simulink model "Control_test"  (R2014b)
settings: Solver=FixedStepDiscrete  StartTime=0.0  StopTime=Inf  FixedStep=0.001  RelTol=1e-3
PostLoadFcn:
  | , if any(exist('dsrtsu_mdlpostloadfcn', 'file') == [2, 3, 6]), try dsrtsu_mdlpostloadfcn('Execute', bdroot); catch fprintf('Error in PostLoadFcn (dsrtsu_mdlpostloadfcn) for model "%s":\n %s\n', bdroot, lasterr); end, end,
undefined symbols (not defined in the file or in its folder): dtLocal, slcm
libraries: rtican x163, simulink x14
(part 30 of 34)

== system Control_test/InputProcessing/RadarCanProcessing/Track64 ==
  Bus Creator : BusCreator  Inputs=12
  ESR_Track64 : rtican/RTICAN Receive (RX)   Reserved1=[]  Reserved2=[]  Reserved3=[]  Reserved4=[]  SfcnMessage=[]  Msg_Struct=[]  BoardTypeNo=[]  BoardNo=[]  ChannelNo=[]  Parameters=[]  DialogFcn=[]  UnitName=[]  Revision=[]  UnitValues=[]  DSProperties=struct('RTI',struct('Version',uint32(5),'BlockType',struct('isSLSource',uint8(1),'isSLSink',uint8(1),'isHWSource',uint8(0),'isHWSink',uint8(0),'isSetup',uint8(0),'isInline',uint8(1),'isNonInline',uint8(0),'isInterrupt',uint8(0),'isChannelwise',uint8(0)),'IOBoardType','RTICAN','UnitType','MESSAGE','Identifier','RX','DialogType','MSVC','BlockSet','RTICAN','SlaveProcessor','CAN'))  RTIBlockInterface=struct('OutputPortsWidth',int32([1 1 1 1 1 1 1 1 1 1 1 1]),'OutputPortsActive',[1 1 1 1 1 1 1 1 1 1 1 1],'OutputPortsName',{{'CAN_TX_TRACK_RANGE_RATE_64','CAN_TX_TRACK_MED_RANGE_MODE_64','CAN_TX_TRACK_RANGE_ACCEL_64','CAN_TX_TRACK_WIDTH_64','CAN_TX_TRACK_ROLLING_COUNT_64','CAN_TX_TRACK_BRIDGE_OBJECT_64','CAN_TX_TRACK_RANGE_64','CAN_TX_TRACK_ANGLE_64','CAN_TX_TRACK_STATUS_64','CAN_TX_TRACK_ONCOMING_64','CAN_TX_TRACK_GROUPING_CHANGED_64','CAN_TX_TRACK_LAT_RATE_64'}},'OutputPortsDataType',{{'SS_DOUBLE','SS_DOUBLE','SS_DOUBLE','SS_DOUBLE','SS_DOUBLE','SS_DOUBLE','SS_DOUBLE','SS_DOUBLE','SS_DOUBLE','SS_DOUBLE','SS_DOUBLE','SS_DOUBLE'}},'OutputPortsLabel',{{'CAN_TX_TRACK_RANGE_RATE_64','CAN_TX_TRACK_MED_RANGE_MODE_64','CAN_TX_TRACK_RANGE_ACCEL_64','CAN_TX_TRACK_WIDTH_64','CAN_TX_TRACK_ROLLING_COUNT_64','CAN_TX_TRACK_BRIDGE_OBJECT_64','CAN_TX_TRACK_RANGE_64','CAN_TX_TRACK_ANGLE_64','CAN_TX_TRACK_STATUS_64','CAN_TX_TRACK_ONCOMING_64','CAN_TX_TRACK_GROUPING_CHANGED_64','CAN_TX_TRACK_LAT_RATE_64'}},'OutputPortsLabelMode','ON','InputPortsWidth',int32(0),'InputPortsActive',0,'DialogFcn','rtican_message_interface_gui','BlockDisplay',{{'','center'}},'IconTransparency','on','ParameterTunableNames',{{}},'InitLevel',3,'BlockName',struct('Token',{{'ESR_Track64'}}),'SampleTime',{{0.01}},'TriggerPort',{{'none'}},'EnablePort',{{'none'}})  RTIBlockParameters=struct('BoardTypeNo',{{1,'OFF',[]}},'BoardNo',{{2,'ON',[1 16]}},'ChannelNo',{{2,'ON',[1 2]}},'Parameters',{{struct('DataFileSupport',struct('DataFileSelectedMaster',1,'DataFileSelectedLocal',0,'DataFileName','c:\users\mpc_car\documents\github\mpc-car\controller\dbcfiles\esr_dv3_64tgt.dbc|','DataFileDate',{{{['02-Nov-2012 20:32:52']},{['21-Mar-2013 13:39:53']},{['28-Sep-2011 17:08:52']}}},'SelectedFile',['<no file selected>'],'InterfaceFcn','rtican_dbc_file_parser'),'Options',struct('StatusSelected',0,'TimeSelected',0,'DeltaTimeSelected',0,'BytePortSelected',0,'MessageLengthSelected',0,'TriggerPort',struct('Selected',0,'TriggerType',0),'UserCoding',struct('Selected',0,'InterfaceFile','UserDecodingFile','FcnName','UserDecodeFcn','InportSelected',0,'InportWidth',1,'OutportSelected',0,'OutportWidth',1),'EnablePortSelected',0,'SignalOnPortnameSelected',1,'UseRXService',0),'Message',struct('MsgOnBlocknameSelected',1,'MsgName','ESR_Track64','MsgIdFormat',0,'MsgId',1343,'MsgLength',8,'NumSignals',12,'SampleTime',0.01,'Signal',struct('SgnName',{'CAN_TX_TRACK_RANGE_RATE_64','CAN_TX_TRACK_MED_RANGE_MODE_64','CAN_TX_TRACK_RANGE_ACCEL_64','CAN_TX_TRACK_WIDTH_64','CAN_TX_TRACK_ROLLING_COUNT_64','CAN_TX_TRACK_BRIDGE_OBJECT_64','CAN_TX_TRACK_RANGE_64','CAN_TX_TRACK_ANGLE_64','CAN_TX_TRACK_STATUS_64','CAN_TX_TRACK_ONCOMING_64','CAN_TX_TRACK_GROUPING_CHANGED_64','CAN_TX_TRACK_LAT_RATE_64'},'SgnStartBit',{0,14,16,26,30,31,32,43,53,56,57,58},'SgnLength',{14,2,10,4,1,1,11,10,3,1,1,6},'SgnType',{0,0,0,0,0,0,0,0,0,0,0,0},'ModeValue',{-1,-1,-1,-1,-1,-1,-1,-1,-1,-1,-1,-1},'DataType',{1,0,1,0,0,0,0,1,0,0,0,1},'ByteLayout',{2,2,2,2,2,2,2,2,2,2,2,2},'Factor',{0.01,1,0.05,0.5,1,1,0.1,0.1,1,1,1,0.25},'Offset',{0,0,0,0,0,0,0,0,0,0,0,0},'SgnComment',{{''},{''},{''},{''},{''},{''},{''},{''},{''},{''},{''},{''}},'SgnUnit',{'m/s','','m/s/s','m','','','m','deg','','','',''},'Min',{-81.92,0,-25.6,0,0,0,0,-51.2,0,0,0,-8},'Max',{81.91,3,25.55,7.5,1,0,204.7,51.1,7,0,0,7.75},'SLDataType',{'SS_DOUBLE','SS_DOUBLE','SS_DOUBLE','SS_DOUBLE','SS_DOUBLE','SS_DOUBLE','SS_DOUBLE','SS_DOUBLE','SS_DOUBLE','SS_DOUBLE','SS_DOUBLE','SS_DOUBLE'}),'MsgIdNumFormat',0,'MsgComment',{{''}}),'Version',1.2,'general',struct('isFromLib',0)),'OFF',[]}},'GroupId',{{struct('Group',{{'RTICAN'}},'No',4,'Behavior',{{'NAMECHANGE'}},'BlockType',{{'SINK'}},'NameChangeFlag',0),'OFF',[]}},'SFcnRTICANMessage',{{struct('MsgType','RX','SFcnPortType','Scalar','MsgName','ESR_Track64','MsgIdFormat','STD','MsgId',1343,'MsgLength',8,'NumSignals',12,'SampleTime',0.01,'Signal',struct('SgnName',{'CAN_TX_TRACK_RANGE_RATE_64','CAN_TX_TRACK_MED_RANGE_MODE_64','CAN_TX_TRACK_RANGE_ACCEL_64','CAN_TX_TRACK_WIDTH_64','CAN_TX_TRACK_ROLLING_COUNT_64','CAN_TX_TRACK_BRIDGE_OBJECT_64','CAN_TX_TRACK_RANGE_64','CAN_TX_TRACK_ANGLE_64','CAN_TX_TRACK_STATUS_64','CAN_TX_TRACK_ONCOMING_64','CAN_TX_TRACK_GROUPING_CHANGED_64','CAN_TX_TRACK_LAT_RATE_64'},'SgnStartBit',{0,14,16,26,30,31,32,43,53,56,57,58},'SgnLength',{14,2,10,4,1,1,11,10,3,1,1,6},'SgnType',{'standard','standard','standard','standard','standard','standard','standard','standard','standard','standard','standard','standard'},'ModeValue',{-1,-1,-1,-1,-1,-1,-1,-1,-1,-1,-1,-1},'DataType',{['signed int'],['unsigned int'],['signed int'],['unsigned int'],['unsigned int'],['unsigned int'],['unsigned int'],['signed int'],['unsigned int'],['unsigned int'],['unsigned int'],['signed int']},'ByteLayout',{['motorola back.'],['motorola back.'],['motorola back.'],['motorola back.'],['motorola back.'],['motorola back.'],['motorola back.'],['motorola back.'],['motorola back.'],['motorola back.'],['motorola back.'],['motorola back.']},'Factor',{0.01,1,0.05,0.5,1,1,0.1,0.1,1,1,1,0.25},'Offset',{0,0,0,0,0,0,0,0,0,0,0,0},'SLDataType',{'SS_DOUBLE','SS_DOUBLE','SS_DOUBLE','SS_DOUBLE','SS_DOUBLE','SS_DOUBLE','SS_DOUBLE','SS_DOUBLE','SS_DOUBLE','SS_DOUBLE','SS_DOUBLE','SS_DOUBLE'}),'StatusSelected','no','TimeSelected','no','DeltaTimeSelected','no','BytePortSelected','no','MessageLengthSelected','no','TriggerPort',struct('Selected','no','TriggerType',0),'UserCoding',struct('Selected','no','InterfaceFile','UserDecodingFile','FcnName','UserDecodeFcn','InportSelected','no','InportWidth',1,'OutportSelected','no','OutportWidth',1),'EnablePortSelected','no','UseRXService','no','BoardType','DS1','BoardNo',2,'ControllerNo',2),'OFF',[]}},'TLCFileName',{{'rtican_rx_message','OFF',[]}})  RTISFcnParameters=struct('SFcnRTICANMessage','struct','TLCFileName','char')  RTIBlockParaDefault=struct('BoardTypeNo',4302,'BoardNo',1,'ChannelNo',1,'Parameters',struct('DataFileSupport',struct('DataFileSelectedMaster',0,'DataFileSelectedLocal',0,'DataFileName','','DataFileDate','','SelectedFile',['<no file selected>']),'Options',struct('StatusSelected',1,'TimeSelected',1,'DeltaTimeSelected',1,'BytePortSelected',0,'MessageLengthSelected',0,'TriggerPort',struct('Selected',0,'TriggerType','rising'),'UserCoding',struct('Selected',0,'InterfaceFile','UserDecodingFile','FcnName','UserDecodeFcn','InportSelected',0,'InportWidth',1,'OutportSelected',0,'OutportWidth',1),'EnablePortSelected',0,'SignalOnPortnameSelected',1,'UseRXService',0),'Message',struct('MsgOnBlocknameSelected',0,'MsgName',['RX Message'],'MsgIdFormat',0,'MsgId',100,'MsgLength',8,'NumSignals',1,'SampleTime',-1,'Signal',struct('SgnName',['RX signal'],'SgnStartBit',0,'SgnLength',8,'SgnType',0,'ModeValue',-1,'DataType',0,'SLDataType','SS_DOUBLE','ByteLayout',0,'Factor',1,'Offset',0,'Min',0,'Max',255,'SgnComment',{{}},'SgnUnit',''),'MsgIdNumFormat',0,'MsgComment',{{''}}),'Version',1.2,'general',struct('isFromLib',1)),'GroupId',struct('Group',{{'RTICAN'}},'No',1,'Behavior',{{'NAMECHANGE'}},'BlockType',{{'SINK'}},'NameChangeFlag',0),'SFcnRTICANMessage',struct('MsgType','RX','MsgName',['RX Message'],'MsgIdFormat','STD','MsgId',100,'MsgLength',8,'NumSignals',1,'SampleTime',-1,'Signal',struct('SgnName',['RX signal'],'SgnStartBit',0,'SgnLength',8,'SgnType','standard','ModeValue',-1,'DataType',['unsigned int'],'ByteLayout',['little endian'],'SLDataType','SS_DOUBLE','Factor',1,'Offset',0),'StatusSelected','yes','TimeSelected','yes','DeltaTimeSelected','yes','BytePortSelected','no','MessageLengthSelected','no','EnablePortSelected','no','UserCoding',struct('Selected','no','InterfaceFile','UserDecodingFile','FcnName','UserDecodeFcn','InportSelected','no','InportWidth',1,'OutportSelected','no','OutportWidth',1),'TriggerPort',struct('Selected','no','TriggerType','rising'),'UseRXService','no','BoardType','DS4302','BoardNo',1,'ControllerNo',1,'SFcnPortType','Scalar'),'TLCFileName','rtican_rx_message')
      settings: AttributesFormatString=Group Id: RTICAN4\n
  Out1 : Outport
  wires:
  Bus Creator/1 -> Out1/1  "Track64"
  ESR_Track64/1 -> Bus Creator/1  "CAN_TX_TRACK_RANGE_RATE_64"
  ESR_Track64/2 -> Bus Creator/2  "CAN_TX_TRACK_MED_RANGE_MODE_64"
  ESR_Track64/3 -> Bus Creator/3  "CAN_TX_TRACK_RANGE_ACCEL_64"
  ESR_Track64/4 -> Bus Creator/4  "CAN_TX_TRACK_WIDTH_64"
  ESR_Track64/5 -> Bus Creator/5  "CAN_TX_TRACK_ROLLING_COUNT_64"
  ESR_Track64/6 -> Bus Creator/6  "CAN_TX_TRACK_BRIDGE_OBJECT_64"
  ESR_Track64/7 -> Bus Creator/7  "CAN_TX_TRACK_RANGE_64"
  ESR_Track64/8 -> Bus Creator/8  "CAN_TX_TRACK_ANGLE_64"
  ESR_Track64/9 -> Bus Creator/9  "CAN_TX_TRACK_STATUS_64"
  ESR_Track64/10 -> Bus Creator/10  "CAN_TX_TRACK_ONCOMING_64"
  ESR_Track64/11 -> Bus Creator/11  "CAN_TX_TRACK_GROUPING_CHANGED_64"
  ESR_Track64/12 -> Bus Creator/12  "CAN_TX_TRACK_LAT_RATE_64"

== system Control_test/InputProcessing/VehicleCanProcessing/CLU1 ==
  Bus Creator : BusCreator  Inputs=15
  L_CLU1 : rtican/RTICAN Receive (RX)   Reserved1=[]  Reserved2=[]  Reserved3=[]  Reserved4=[]  SfcnMessage=[]  Msg_Struct=[]  BoardTypeNo=[]  BoardNo=[]  ChannelNo=[]  Parameters=[]  DialogFcn=[]  UnitName=[]  Revision=[]  UnitValues=[]  DSProperties=struct('RTI',struct('Version',uint32(5),'BlockType',struct('isSLSource',uint8(1),'isSLSink',uint8(1),'isHWSource',uint8(0),'isHWSink',uint8(0),'isSetup',uint8(0),'isInline',uint8(1),'isNonInline',uint8(0),'isInterrupt',uint8(0),'isChannelwise',uint8(0)),'IOBoardType','RTICAN','UnitType','MESSAGE','Identifier','RX','DialogType','MSVC','BlockSet','RTICAN','SlaveProcessor','CAN'))  RTIBlockInterface=struct('OutputPortsWidth',int32([1 1 1 1 1 1 1 1 1 1 1 1 1 1 1]),'OutputPortsActive',[1 1 1 1 1 1 1 1 1 1 1 1 1 1 1],'OutputPortsName',{{'CruiseSWStatus','CF_Blr_MaxStat','CF_Clu_SldMainSW','SPEED_UNIT','P_Brake_ACT','Vanz','AliveCounter','CruiseSW_Main','DashACCFail','DISFail','VEHICLE_INFO','CF_StrRly_Stat','CF_ButSys_VarInd','R_TqAcnOutC','Odometer'}},'OutputPortsDataType',{{'SS_DOUBLE','SS_DOUBLE','SS_DOUBLE','SS_DOUBLE','SS_DOUBLE','SS_DOUBLE','SS_DOUBLE','SS_DOUBLE','SS_DOUBLE','SS_DOUBLE','SS_DOUBLE','SS_DOUBLE','SS_DOUBLE','SS_DOUBLE','SS_DOUBLE'}},'OutputPortsLabel',{{'CruiseSWStatus','CF_Blr_MaxStat','CF_Clu_SldMainSW','SPEED_UNIT','P_Brake_ACT','Vanz','AliveCounter','CruiseSW_Main','DashACCFail','DISFail','VEHICLE_INFO','CF_StrRly_Stat','CF_ButSys_VarInd','R_TqAcnOutC','Odometer'}},'OutputPortsLabelMode','ON','InputPortsWidth',int32(0),'InputPortsActive',0,'DialogFcn','rtican_message_interface_gui','BlockDisplay',{{'','center'}},'IconTransparency','on','ParameterTunableNames',{{}},'InitLevel',3,'BlockName',struct('Token',{{'L_CLU1'}}),'SampleTime',{{-1}},'TriggerPort',{{'none'}},'EnablePort',{{'none'}})  RTIBlockParameters=struct('BoardTypeNo',{{1,'OFF',[]}},'BoardNo',{{1,'ON',[1 16]}},'ChannelNo',{{1,'ON',[1 2]}},'Parameters',{{struct('DataFileSupport',struct('DataFileSelectedMaster',1,'DataFileSelectedLocal',1,'DataFileName','c:\users\mpc_car\documents\github\mpc-car\controller\dbcfiles\hmc_can_for_ucb_v2.dbc|','DataFileDate',{{{['21-Nov-2014 13:30:51']}}},'SelectedFile','c:\users\mpc_car\documents\github\mpc-car\dbcfiles\hmc_can_for_ucb_v2.dbc','InterfaceFcn','rtican_dbc_file_parser'),'Options',struct('StatusSelected',0,'TimeSelected',0,'DeltaTimeSelected',0,'BytePortSelected',0,'MessageLengthSelected',0,'TriggerPort',struct('Selected',0,'TriggerType',0),'UserCoding',struct('Selected',0,'InterfaceFile','UserDecodingFile','FcnName','UserDecodeFcn','InportSelected',0,'InportWidth',1,'OutportSelected',0,'OutportWidth',1),'EnablePortSelected',0,'SignalOnPortnameSelected',1,'UseRXService',0),'Message',struct('MsgOnBlocknameSelected',1,'MsgName','L_CLU1','MsgIdFormat',0,'MsgId',1264,'MsgLength',8,'NumSignals',15,'SampleTime',-1,'Signal',struct('SgnName',{'CruiseSWStatus','CF_Blr_MaxStat','CF_Clu_SldMainSW','SPEED_UNIT','P_Brake_ACT','Vanz','AliveCounter','CruiseSW_Main','DashACCFail','DISFail','VEHICLE_INFO','CF_StrRly_Stat','CF_ButSys_VarInd','R_TqAcnOutC','Odometer'},'SgnStartBit',{0,3,4,6,7,8,17,24,25,26,27,30,31,32,40},'SgnLength',{3,1,1,1,1,9,7,1,1,1,3,1,1,8,24},'SgnType',{0,0,0,0,0,0,0,0,0,0,0,0,0,0,0},'ModeValue',{-1,-1,-1,-1,-1,-1,-1,-1,-1,-1,-1,-1,-1,-1,-1},'DataType',{0,0,0,0,0,0,0,0,0,0,0,0,0,0,0},'ByteLayout',{0,0,0,0,0,0,0,0,0,0,0,0,0,0,0},'Factor',{1,1,1,1,1,1,1,1,1,1,1,1,1,1,1},'Offset',{0,0,0,0,0,0,0,0,0,0,0,0,0,0,0},'SgnComment',{{''},{''},{''},{''},{''},{''},{''},{''},{''},{''},{''},{''},{''},{''},{''}},'SgnUnit',{'','','','','',['km/h or MPH'],'','','','','','','','Nm','km'},'Min',{0,0,0,0,0,0,0,0,0,0,0,0,0,0,0},'Max',{7,1,1,1,1,255.5,127,1,1,1,7,1,1,255,1677721.5},'SLDataType',{'SS_DOUBLE','SS_DOUBLE','SS_DOUBLE','SS_DOUBLE','SS_DOUBLE','SS_DOUBLE','SS_DOUBLE','SS_DOUBLE','SS_DOUBLE','SS_DOUBLE','SS_DOUBLE','SS_DOUBLE','SS_DOUBLE','SS_DOUBLE','SS_DOUBLE'}),'MsgIdNumFormat',0,'MsgComment',{{''}}),'Version',1.2,'general',struct('isFromLib',0)),'OFF',[]}},'GroupId',{{struct('Group',{{'RTICAN'}},'No',1,'Behavior',{{'NAMECHANGE'}},'BlockType',{{'SINK'}},'NameChangeFlag',0),'OFF',[]}},'SFcnRTICANMessage',{{struct('MsgType','RX','SFcnPortType','Scalar','MsgName','L_CLU1','MsgIdFormat','STD','MsgId',1264,'MsgLength',8,'NumSignals',15,'SampleTime',-1,'Signal',struct('SgnName',{'CruiseSWStatus','CF_Blr_MaxStat','CF_Clu_SldMainSW','SPEED_UNIT','P_Brake_ACT','Vanz','AliveCounter','CruiseSW_Main','DashACCFail','DISFail','VEHICLE_INFO','CF_StrRly_Stat','CF_ButSys_VarInd','R_TqAcnOutC','Odometer'},'SgnStartBit',{0,3,4,6,7,8,17,24,25,26,27,30,31,32,40},'SgnLength',{3,1,1,1,1,9,7,1,1,1,3,1,1,8,24},'SgnType',{'standard','standard','standard','standard','standard','standard','standard','standard','standard','standard','standard','standard','standard','standard','standard'},'ModeValue',{-1,-1,-1,-1,-1,-1,-1,-1,-1,-1,-1,-1,-1,-1,-1},'DataType',{['unsigned int'],['unsigned int'],['unsigned int'],['unsigned int'],['unsigned int'],['unsigned int'],['unsigned int'],['unsigned int'],['unsigned int'],['unsigned int'],['unsigned int'],['unsigned int'],['unsigned int'],['unsigned int'],['unsigned int']},'ByteLayout',{['little endian'],['little endian'],['little endian'],['little endian'],['little endian'],['little endian'],['little endian'],['little endian'],['little endian'],['little endian'],['little endian'],['little endian'],['little endian'],['little endian'],['little endian']},'Factor',{1,1,1,1,1,1,1,1,1,1,1,1,1,1,1},'Offset',{0,0,0,0,0,0,0,0,0,0,0,0,0,0,0},'SLDataType',{'SS_DOUBLE','SS_DOUBLE','SS_DOUBLE','SS_DOUBLE','SS_DOUBLE','SS_DOUBLE','SS_DOUBLE','SS_DOUBLE','SS_DOUBLE','SS_DOUBLE','SS_DOUBLE','SS_DOUBLE','SS_DOUBLE','SS_DOUBLE','SS_DOUBLE'}),'StatusSelected','no','TimeSelected','no','DeltaTimeSelected','no','BytePortSelected','no','MessageLengthSelected','no','TriggerPort',struct('Selected','no','TriggerType',0),'UserCoding',struct('Selected','no','InterfaceFile','UserDecodingFile','FcnName','UserDecodeFcn','InportSelected','no','InportWidth',1,'OutportSelected','no','OutportWidth',1),'EnablePortSelected','no','UseRXService','no','BoardType','DS1','BoardNo',1,'ControllerNo',1),'OFF',[]}},'TLCFileName',{{'rtican_rx_message','OFF',[]}})  RTISFcnParameters=struct('SFcnRTICANMessage','struct','TLCFileName','char')  RTIBlockParaDefault=struct('BoardTypeNo',4302,'BoardNo',1,'ChannelNo',1,'Parameters',struct('DataFileSupport',struct('DataFileSelectedMaster',0,'DataFileSelectedLocal',0,'DataFileName','','DataFileDate','','SelectedFile',['<no file selected>']),'Options',struct('StatusSelected',1,'TimeSelected',1,'DeltaTimeSelected',1,'BytePortSelected',0,'MessageLengthSelected',0,'TriggerPort',struct('Selected',0,'TriggerType','rising'),'UserCoding',struct('Selected',0,'InterfaceFile','UserDecodingFile','FcnName','UserDecodeFcn','InportSelected',0,'InportWidth',1,'OutportSelected',0,'OutportWidth',1),'EnablePortSelected',0,'SignalOnPortnameSelected',1,'UseRXService',0),'Message',struct('MsgOnBlocknameSelected',0,'MsgName',['RX Message'],'MsgIdFormat',0,'MsgId',100,'MsgLength',8,'NumSignals',1,'SampleTime',-1,'Signal',struct('SgnName',['RX signal'],'SgnStartBit',0,'SgnLength',8,'SgnType',0,'ModeValue',-1,'DataType',0,'SLDataType','SS_DOUBLE','ByteLayout',0,'Factor',1,'Offset',0,'Min',0,'Max',255,'SgnComment',{{}},'SgnUnit',''),'MsgIdNumFormat',0,'MsgComment',{{''}}),'Version',1.2,'general',struct('isFromLib',1)),'GroupId',struct('Group',{{'RTICAN'}},'No',1,'Behavior',{{'NAMECHANGE'}},'BlockType',{{'SINK'}},'NameChangeFlag',0),'SFcnRTICANMessage',struct('MsgType','RX','MsgName',['RX Message'],'MsgIdFormat','STD','MsgId',100,'MsgLength',8,'NumSignals',1,'SampleTime',-1,'Signal',struct('SgnName',['RX signal'],'SgnStartBit',0,'SgnLength',8,'SgnType','standard','ModeValue',-1,'DataType',['unsigned int'],'ByteLayout',['little endian'],'SLDataType','SS_DOUBLE','Factor',1,'Offset',0),'StatusSelected','yes','TimeSelected','yes','DeltaTimeSelected','yes','BytePortSelected','no','MessageLengthSelected','no','EnablePortSelected','no','UserCoding',struct('Selected','no','InterfaceFile','UserDecodingFile','FcnName','UserDecodeFcn','InportSelected','no','InportWidth',1,'OutportSelected','no','OutportWidth',1),'TriggerPort',struct('Selected','no','TriggerType','rising'),'UseRXService','no','BoardType','DS4302','BoardNo',1,'ControllerNo',1,'SFcnPortType','Scalar'),'TLCFileName','rtican_rx_message')
      settings: AttributesFormatString=Group Id: RTICAN1\n
  CLU1_CAN : Outport
  tag scope: CruiseSWStatus=global, CruiseSW_Main=global
  wires:
  Bus Creator/1 -> CLU1_CAN/1  "CLU1_CAN"
  L_CLU1/1 -> Bus Creator/1, [CruiseSWStatus]  "CruiseSWStatus"
  L_CLU1/2 -> Bus Creator/2  "CF_Blr_MaxStat"
  L_CLU1/3 -> Bus Creator/3  "CF_Clu_SldMainSW"
  L_CLU1/4 -> Bus Creator/4  "SPEED_UNIT"
  L_CLU1/5 -> Bus Creator/5  "P_Brake_ACT"
  L_CLU1/6 -> Bus Creator/6  "Vanz"
  L_CLU1/7 -> Bus Creator/7  "AliveCounter"
  L_CLU1/8 -> [CruiseSW_Main], Bus Creator/8  "CruiseSW_Main"
  L_CLU1/9 -> Bus Creator/9  "DashACCFail"
  L_CLU1/10 -> Bus Creator/10  "DISFail"
  L_CLU1/11 -> Bus Creator/11  "VEHICLE_INFO"
  L_CLU1/12 -> Bus Creator/12  "CF_StrRly_Stat"
  L_CLU1/13 -> Bus Creator/13  "CF_ButSys_VarInd"
  L_CLU1/14 -> Bus Creator/14  "R_TqAcnOutC"
  L_CLU1/15 -> Bus Creator/15  "Odometer"

== system Control_test/InputProcessing/VehicleCanProcessing/CLU1Processing ==
  In1 : Inport
  Out1 : Outport
  wires:
  In1/1 -> Out1/1  "CLU1Data"

== system Control_test/InputProcessing/VehicleCanProcessing/CLU2 ==
  Bus Creator : BusCreator  Inputs=31
  L_CLU2 : rtican/RTICAN Receive (RX)   Reserved1=[]  Reserved2=[]  Reserved3=[]  Reserved4=[]  SfcnMessage=[]  Msg_Struct=[]  BoardTypeNo=[]  BoardNo=[]  ChannelNo=[]  Parameters=[]  DialogFcn=[]  UnitName=[]  Revision=[]  UnitValues=[]  DSProperties=struct('RTI',struct('Version',uint32(5),'BlockType',struct('isSLSource',uint8(1),'isSLSink',uint8(1),'isHWSource',uint8(0),'isHWSink',uint8(0),'isSetup',uint8(0),'isInline',uint8(1),'isNonInline',uint8(0),'isInterrupt',uint8(0),'isChannelwise',uint8(0)),'IOBoardType','RTICAN','UnitType','MESSAGE','Identifier','RX','DialogType','MSVC','BlockSet','RTICAN','SlaveProcessor','CAN'))  RTIBlockInterface=struct('OutputPortsWidth',int32([1 1 1 1 1 1 1 1 1 1 1 1 1 1 1 1 1 1 1 1 1 1 1 1 1 1 1 1 1 1 1]),'OutputPortsActive',[1 1 1 1 1 1 1 1 1 1 1 1 1 1 1 1 1 1 1 1 1 1 1 1 1 1 1 1 1 1 1],'OutputPortsName',{{'DRV_DR_SW','PIC_Lock','DRV_Key_Lock','CF_Clu_LkasDispMode','CF_Clu_HeadLampHigh','CF_Clu_AltLStatus','PIC_Unlock','CF_Clu_WiperIntT','DRV_Seat_Belt','TRUNK_OPEN_STATUS','PAS_Seat_Belt','CF_HoodStat','CF_Clu_TurnSigLh','CF_Clu_TurnSigRh','CF_Clu_LdwsLkasSW','CF_Clu_SwiGearR','CF_Clu_EcoDriveInf','CF_Clu_WiperHigh','CF_Clu_WiperAuto','CF_Clu_RainSnsStat','CF_Clu_HazardSW','CF_Clu_ActiveEcoSW','DRV_Key_Unlock','CF_Clu_WiperIntSW','CF_Clu_WiperLow','CF_SWL_Stat','AST_DR_SW','CF_Clu_HeadLampLow','IGN_SW','RKE_CMD','CF_Clu_AliveCnt2'}},'OutputPortsDataType',{{'SS_DOUBLE','SS_DOUBLE','SS_DOUBLE','SS_DOUBLE','SS_DOUBLE','SS_DOUBLE','SS_DOUBLE','SS_DOUBLE','SS_DOUBLE','SS_DOUBLE','SS_DOUBLE','SS_DOUBLE','SS_DOUBLE','SS_DOUBLE','SS_DOUBLE','SS_DOUBLE','SS_DOUBLE','SS_DOUBLE','SS_DOUBLE','SS_DOUBLE','SS_DOUBLE','SS_DOUBLE','SS_DOUBLE','SS_DOUBLE','SS_DOUBLE','SS_DOUBLE','SS_DOUBLE','SS_DOUBLE','SS_DOUBLE','SS_DOUBLE','SS_DOUBLE'}},'OutputPortsLabel',{{'DRV_DR_SW','PIC_Lock','DRV_Key_Lock','CF_Clu_LkasDispMode','CF_Clu_HeadLampHigh','CF_Clu_AltLStatus','PIC_Unlock','CF_Clu_WiperIntT','DRV_Seat_Belt','TRUNK_OPEN_STATUS','PAS_Seat_Belt','CF_HoodStat','CF_Clu_TurnSigLh','CF_Clu_TurnSigRh','CF_Clu_LdwsLkasSW','CF_Clu_SwiGearR','CF_Clu_EcoDriveInf','CF_Clu_WiperHigh','CF_Clu_WiperAuto','CF_Clu_RainSnsStat','CF_Clu_HazardSW','CF_Clu_ActiveEcoSW','DRV_Key_Unlock','CF_Clu_WiperIntSW','CF_Clu_WiperLow','CF_SWL_Stat','AST_DR_SW','CF_Clu_HeadLampLow','IGN_SW','RKE_CMD','CF_Clu_AliveCnt2'}},'OutputPortsLabelMode','ON','InputPortsWidth',int32(0),'InputPortsActive',0,'DialogFcn','rtican_message_interface_gui','BlockDisplay',{{'','center'}},'IconTransparency','on','ParameterTunableNames',{{}},'InitLevel',3,'BlockName',struct('Token',{{'L_CLU2'}}),'SampleTime',{{-1}},'TriggerPort',{{'none'}},'EnablePort',{{'none'}})  RTIBlockParameters=struct('BoardTypeNo',{{1,'OFF',[]}},'BoardNo',{{1,'ON',[1 16]}},'ChannelNo',{{1,'ON',[1 2]}},'Parameters',{{struct('DataFileSupport',struct('DataFileSelectedMaster',1,'DataFileSelectedLocal',1,'DataFileName','c:\users\mpc_car\documents\github\mpc-car\controller\dbcfiles\hmc_can_for_ucb_v2.dbc|','DataFileDate',['21-Nov-2014 13:30:51'],'SelectedFile','c:\users\mpc_car\documents\github\mpc-car\dbcfiles\hmc_can_for_ucb_v2.dbc','InterfaceFcn','rtican_dbc_file_parser'),'Options',struct('StatusSelected',0,'TimeSelected',0,'DeltaTimeSelected',0,'BytePortSelected',0,'MessageLengthSelected',0,'TriggerPort',struct('Selected',0,'TriggerType',0),'UserCoding',struct('Selected',0,'InterfaceFile','UserDecodingFile','FcnName','UserDecodeFcn','InportSelected',0,'InportWidth',1,'OutportSelected',0,'OutportWidth',1),'EnablePortSelected',0,'SignalOnPortnameSelected',1,'UseRXService',0),'Message',struct('MsgOnBlocknameSelected',1,'MsgName','L_CLU2','MsgIdFormat',0,'MsgId',513,'MsgLength',8,'NumSignals',31,'SampleTime',-1,'Signal',struct('SgnName',{'DRV_DR_SW','PIC_Lock','DRV_Key_Lock','CF_Clu_LkasDispMode','CF_Clu_HeadLampHigh','CF_Clu_AltLStatus','PIC_Unlock','CF_Clu_WiperIntT','DRV_Seat_Belt','TRUNK_OPEN_STATUS','PAS_Seat_Belt','CF_HoodStat','CF_Clu_TurnSigLh','CF_Clu_TurnSigRh','CF_Clu_LdwsLkasSW','CF_Clu_SwiGearR','CF_Clu_EcoDriveInf','CF_Clu_WiperHigh','CF_Clu_WiperAuto','CF_Clu_RainSnsStat','CF_Clu_HazardSW','CF_Clu_ActiveEcoSW','DRV_Key_Unlock','CF_Clu_WiperIntSW','CF_Clu_WiperLow','CF_SWL_Stat','AST_DR_SW','CF_Clu_HeadLampLow','IGN_SW','RKE_CMD','CF_Clu_AliveCnt2'},'SgnStartBit',{0,2,5,6,8,9,10,13,16,18,20,22,24,25,26,27,29,32,33,34,37,38,39,40,41,42,45,47,48,51,56},'SgnLength',{2,3,1,2,1,1,3,3,2,2,2,2,1,1,1,2,3,1,1,3,1,1,1,1,1,3,2,1,3,3,4},'ByteLayout',{0,0,0,0,0,0,0,0,0,0,0,0,0,0,0,0,0,0,0,0,0,0,0,0,0,0,0,0,0,0,0},'Factor',{1,1,1,1,1,1,1,1,1,1,1,1,1,1,1,1,1,1,1,1,1,1,1,1,1,1,1,1,1,1,1},'Offset',{0,0,0,0,0,0,0,0,0,0,0,0,0,0,0,0,0,0,0,0,0,0,0,0,0,0,0,0,0,0,0},'SgnComment',{'','','','','','','','','','','','','','','','','','','','','',['This signal is for the Active ECO equipped vehicle only.This signal is for the Active ECO equipped vehicle only.'],'','','','','','','','',''},'SgnUnit',{'','','','','','','','','','','','','','','','','','','','','','','','','','','','','','',''},'Min',{0,0,0,0,0,0,0,0,0,0,0,0,0,0,0,0,0,0,0,0,0,0,0,0,0,0,0,0,0,0,0},'Max',{3,7,1,3,1,1,7,7,3,3,3,3,1,1,1,3,7,1,1,7,1,1,1,1,1,7,3,1,7,7,15},'SgnType',{0,0,0,0,0,0,0,0,0,0,0,0,0,0,0,0,0,0,0,0,0,0,0,0,0,0,0,0,0,0,0},'SLDataType',{'SS_DOUBLE','SS_DOUBLE','SS_DOUBLE','SS_DOUBLE','SS_DOUBLE','SS_DOUBLE','SS_DOUBLE','SS_DOUBLE','SS_DOUBLE','SS_DOUBLE','SS_DOUBLE','SS_DOUBLE','SS_DOUBLE','SS_DOUBLE','SS_DOUBLE','SS_DOUBLE','SS_DOUBLE','SS_DOUBLE','SS_DOUBLE','SS_DOUBLE','SS_DOUBLE','SS_DOUBLE','SS_DOUBLE','SS_DOUBLE','SS_DOUBLE','SS_DOUBLE','SS_DOUBLE','SS_DOUBLE','SS_DOUBLE','SS_DOUBLE','SS_DOUBLE'},'DataType',{0,0,0,0,0,0,0,0,0,0,0,0,0,0,0,0,0,0,0,0,0,0,0,0,0,0,0,0,0,0,0},'ModeValue',{-1,-1,-1,-1,-1,-1,-1,-1,-1,-1,-1,-1,-1,-1,-1,-1,-1,-1,-1,-1,-1,-1,-1,-1,-1,-1,-1,-1,-1,-1,-1}),'MsgIdNumFormat',0,'MsgComment',{{''}}),'Version',1.2,'general',struct('isFromLib',0)),'OFF',[]}},'GroupId',{{struct('Group',{{'RTICAN'}},'No',1,'Behavior',{{'NAMECHANGE'}},'BlockType',{{'SINK'}},'NameChangeFlag',0),'OFF',[]}},'SFcnRTICANMessage',{{struct('MsgType','RX','SFcnPortType','Scalar','MsgName','L_CLU2','MsgIdFormat','STD','MsgId',513,'MsgLength',8,'NumSignals',31,'SampleTime',-1,'Signal',struct('SgnName',{'DRV_DR_SW','PIC_Lock','DRV_Key_Lock','CF_Clu_LkasDispMode','CF_Clu_HeadLampHigh','CF_Clu_AltLStatus','PIC_Unlock','CF_Clu_WiperIntT','DRV_Seat_Belt','TRUNK_OPEN_STATUS','PAS_Seat_Belt','CF_HoodStat','CF_Clu_TurnSigLh','CF_Clu_TurnSigRh','CF_Clu_LdwsLkasSW','CF_Clu_SwiGearR','CF_Clu_EcoDriveInf','CF_Clu_WiperHigh','CF_Clu_WiperAuto','CF_Clu_RainSnsStat','CF_Clu_HazardSW','CF_Clu_ActiveEcoSW','DRV_Key_Unlock','CF_Clu_WiperIntSW','CF_Clu_WiperLow','CF_SWL_Stat','AST_DR_SW','CF_Clu_HeadLampLow','IGN_SW','RKE_CMD','CF_Clu_AliveCnt2'},'SgnStartBit',{0,2,5,6,8,9,10,13,16,18,20,22,24,25,26,27,29,32,33,34,37,38,39,40,41,42,45,47,48,51,56},'SgnLength',{2,3,1,2,1,1,3,3,2,2,2,2,1,1,1,2,3,1,1,3,1,1,1,1,1,3,2,1,3,3,4},'ByteLayout',{['little endian'],['little endian'],['little endian'],['little endian'],['little endian'],['little endian'],['little endian'],['little endian'],['little endian'],['little endian'],['little endian'],['little endian'],['little endian'],['little endian'],['little endian'],['little endian'],['little endian'],['little endian'],['little endian'],['little endian'],['little endian'],['little endian'],['little endian'],['little endian'],['little endian'],['little endian'],['little endian'],['little endian'],['little endian'],['little endian'],['little endian']},'Factor',{1,1,1,1,1,1,1,1,1,1,1,1,1,1,1,1,1,1,1,1,1,1,1,1,1,1,1,1,1,1,1},'Offset',{0,0,0,0,0,0,0,0,0,0,0,0,0,0,0,0,0,0,0,0,0,0,0,0,0,0,0,0,0,0,0},'SgnType',{'standard','standard','standard','standard','standard','standard','standard','standard','standard','standard','standard','standard','standard','standard','standard','standard','standard','standard','standard','standard','standard','standard','standard','standard','standard','standard','standard','standard','standard','standard','standard'},'SLDataType',{'SS_DOUBLE','SS_DOUBLE','SS_DOUBLE','SS_DOUBLE','SS_DOUBLE','SS_DOUBLE','SS_DOUBLE','SS_DOUBLE','SS_DOUBLE','SS_DOUBLE','SS_DOUBLE','SS_DOUBLE','SS_DOUBLE','SS_DOUBLE','SS_DOUBLE','SS_DOUBLE','SS_DOUBLE','SS_DOUBLE','SS_DOUBLE','SS_DOUBLE','SS_DOUBLE','SS_DOUBLE','SS_DOUBLE','SS_DOUBLE','SS_DOUBLE','SS_DOUBLE','SS_DOUBLE','SS_DOUBLE','SS_DOUBLE','SS_DOUBLE','SS_DOUBLE'},'DataType',{['unsigned int'],['unsigned int'],['unsigned int'],['unsigned int'],['unsigned int'],['unsigned int'],['unsigned int'],['unsigned int'],['unsigned int'],['unsigned int'],['unsigned int'],['unsigned int'],['unsigned int'],['unsigned int'],['unsigned int'],['unsigned int'],['unsigned int'],['unsigned int'],['unsigned int'],['unsigned int'],['unsigned int'],['unsigned int'],['unsigned int'],['unsigned int'],['unsigned int'],['unsigned int'],['unsigned int'],['unsigned int'],['unsigned int'],['unsigned int'],['unsigned int']},'ModeValue',{-1,-1,-1,-1,-1,-1,-1,-1,-1,-1,-1,-1,-1,-1,-1,-1,-1,-1,-1,-1,-1,-1,-1,-1,-1,-1,-1,-1,-1,-1,-1}),'StatusSelected','no','TimeSelected','no','DeltaTimeSelected','no','BytePortSelected','no','MessageLengthSelected','no','TriggerPort',struct('Selected','no','TriggerType',0),'UserCoding',struct('Selected','no','InterfaceFile','UserDecodingFile','FcnName','UserDecodeFcn','InportSelected','no','InportWidth',1,'OutportSelected','no','OutportWidth',1),'EnablePortSelected','no','UseRXService','no','BoardType','DS1','BoardNo',1,'ControllerNo',1),'OFF',[]}},'TLCFileName',{{'rtican_rx_message','OFF',[]}})  RTISFcnParameters=struct('SFcnRTICANMessage','struct','TLCFileName','char')  RTIBlockParaDefault=struct('BoardTypeNo',4302,'BoardNo',1,'ChannelNo',1,'Parameters',struct('DataFileSupport',struct('DataFileSelectedMaster',0,'DataFileSelectedLocal',0,'DataFileName','','DataFileDate','','SelectedFile',['<no file selected>']),'Options',struct('StatusSelected',1,'TimeSelected',1,'DeltaTimeSelected',1,'BytePortSelected',0,'MessageLengthSelected',0,'TriggerPort',struct('Selected',0,'TriggerType','rising'),'UserCoding',struct('Selected',0,'InterfaceFile','UserDecodingFile','FcnName','UserDecodeFcn','InportSelected',0,'InportWidth',1,'OutportSelected',0,'OutportWidth',1),'EnablePortSelected',0,'SignalOnPortnameSelected',1,'UseRXService',0),'Message',struct('MsgOnBlocknameSelected',0,'MsgName',['RX Message'],'MsgIdFormat',0,'MsgId',100,'MsgLength',8,'NumSignals',1,'SampleTime',-1,'Signal',struct('SgnName',['RX signal'],'SgnStartBit',0,'SgnLength',8,'SgnType',0,'ModeValue',-1,'DataType',0,'SLDataType','SS_DOUBLE','ByteLayout',0,'Factor',1,'Offset',0,'Min',0,'Max',255,'SgnComment',{{}},'SgnUnit',''),'MsgIdNumFormat',0,'MsgComment',{{''}}),'Version',1.2,'general',struct('isFromLib',1)),'GroupId',struct('Group',{{'RTICAN'}},'No',1,'Behavior',{{'NAMECHANGE'}},'BlockType',{{'SINK'}},'NameChangeFlag',0),'SFcnRTICANMessage',struct('MsgType','RX','MsgName',['RX Message'],'MsgIdFormat','STD','MsgId',100,'MsgLength',8,'NumSignals',1,'SampleTime',-1,'Signal',struct('SgnName',['RX signal'],'SgnStartBit',0,'SgnLength',8,'SgnType','standard','ModeValue',-1,'DataType',['unsigned int'],'ByteLayout',['little endian'],'SLDataType','SS_DOUBLE','Factor',1,'Offset',0),'StatusSelected','yes','TimeSelected','yes','DeltaTimeSelected','yes','BytePortSelected','no','MessageLengthSelected','no','EnablePortSelected','no','UserCoding',struct('Selected','no','InterfaceFile','UserDecodingFile','FcnName','UserDecodeFcn','InportSelected','no','InportWidth',1,'OutportSelected','no','OutportWidth',1),'TriggerPort',struct('Selected','no','TriggerType','rising'),'UseRXService','no','BoardType','DS4302','BoardNo',1,'ControllerNo',1,'SFcnPortType','Scalar'),'TLCFileName','rtican_rx_message')
      settings: AttributesFormatString=Group Id: RTICAN1\n
  CLU2_CAN : Outport
  wires:
  Bus Creator/1 -> CLU2_CAN/1  "CLU2_CAN"
  L_CLU2/1 -> Bus Creator/1  "DRV_DR_SW"
  L_CLU2/2 -> Bus Creator/2  "PIC_Lock"
  L_CLU2/3 -> Bus Creator/3  "DRV_Key_Lock"
  L_CLU2/4 -> Bus Creator/4  "CF_Clu_LkasDispMode"
  L_CLU2/5 -> Bus Creator/5  "CF_Clu_HeadLampHigh"
  L_CLU2/6 -> Bus Creator/6  "CF_Clu_AltLStatus"
  L_CLU2/7 -> Bus Creator/7  "PIC_Unlock"
  L_CLU2/8 -> Bus Creator/8  "CF_Clu_WiperIntT"
  L_CLU2/9 -> Bus Creator/9  "DRV_Seat_Belt"
  L_CLU2/10 -> Bus Creator/10  "TRUNK_OPEN_STATUS"
  L_CLU2/11 -> Bus Creator/11  "PAS_Seat_Belt"
  L_CLU2/12 -> Bus Creator/12  "CF_HoodStat"
  L_CLU2/13 -> Bus Creator/13  "CF_Clu_TurnSigLh"
  L_CLU2/14 -> Bus Creator/14  "CF_Clu_TurnSigRh"
  L_CLU2/15 -> Bus Creator/15  "CF_Clu_LdwsLkasSW"
  L_CLU2/16 -> Bus Creator/16  "CF_Clu_SwiGearR"
  L_CLU2/17 -> Bus Creator/17  "CF_Clu_EcoDriveInf"
  L_CLU2/18 -> Bus Creator/18  "CF_Clu_WiperHigh"
  L_CLU2/19 -> Bus Creator/19  "CF_Clu_WiperAuto"
  L_CLU2/20 -> Bus Creator/20  "CF_Clu_RainSnsStat"
  L_CLU2/21 -> Bus Creator/21  "CF_Clu_HazardSW"
  L_CLU2/22 -> Bus Creator/22  "CF_Clu_ActiveEcoSW"
  L_CLU2/23 -> Bus Creator/23  "DRV_Key_Unlock"
  L_CLU2/24 -> Bus Creator/24  "CF_Clu_WiperIntSW"
  L_CLU2/25 -> Bus Creator/25  "CF_Clu_WiperLow"
  L_CLU2/26 -> Bus Creator/26  "CF_SWL_Stat"
  L_CLU2/27 -> Bus Creator/27  "AST_DR_SW"
  L_CLU2/28 -> Bus Creator/28  "CF_Clu_HeadLampLow"
  L_CLU2/29 -> Bus Creator/29  "IGN_SW"
  L_CLU2/30 -> Bus Creator/30  "RKE_CMD"
  L_CLU2/31 -> Bus Creator/31  "CF_Clu_AliveCnt2"

== system Control_test/InputProcessing/VehicleCanProcessing/CLU2Processing ==
  In1 : Inport
  Bus Creator : BusCreator  Inputs=2
  Bus Selector2 : BusSelector  OutputSignals=CF_Clu_TurnSigLh,CF_Clu_TurnSigRh
  CLU2Processing : Subsystem
  Out1 : Outport
  wires:
  Bus Selector2/1 -> CLU2Processing/1(CF_Clu_TrunSigLh_CAN)  "<CF_Clu_TurnSigLh>"
  Bus Selector2/2 -> CLU2Processing/2(CF_Clu_TurnSigRh_CAN)  "<CF_Clu_TurnSigRh>"
  Bus Creator/1 -> Out1/1  "CLU2Data"
  In1/1 -> Bus Selector2/1
  CLU2Processing/1(ipCluTurnSigLh) -> Bus Creator/1
  CLU2Processing/2(ipCluTurnSigRh) -> Bus Creator/2

== system Control_test/InputProcessing/VehicleCanProcessing/EMS1 ==
  Bus Creator : BusCreator  Inputs=13
  L_EMS1 : rtican/RTICAN Receive (RX)   Reserved1=[]  Reserved2=[]  Reserved3=[]  Reserved4=[]  SfcnMessage=[]  Msg_Struct=[]  BoardTypeNo=[]  BoardNo=[]  ChannelNo=[]  Parameters=[]  DialogFcn=[]  UnitName=[]  Revision=[]  UnitValues=[]  DSProperties=struct('RTI',struct('Version',uint32(5),'BlockType',struct('isSLSource',uint8(1),'isSLSink',uint8(1),'isHWSource',uint8(0),'isHWSink',uint8(0),'isSetup',uint8(0),'isInline',uint8(1),'isNonInline',uint8(0),'isInterrupt',uint8(0),'isChannelwise',uint8(0)),'IOBoardType','RTICAN','UnitType','MESSAGE','Identifier','RX','DialogType','MSVC','BlockSet','RTICAN','SlaveProcessor','CAN'))  RTIBlockInterface=struct('OutputPortsWidth',int32([1 1 1 1 1 1 1 1 1 1 1 1 1]),'OutputPortsActive',[1 1 1 1 1 1 1 1 1 1 1 1 1],'OutputPortsName',{{'TQI_ACOR','TQ_COR_STAT','SWI_IGK','ACK_TCS','PUC_STAT','F_N_ENG','RLY_AC','F_SUB_TQI','RATIO_TQI_BAS_MAX_STND','VS','TQI','TQFR','N'}},'OutputPortsDataType',{{'SS_DOUBLE','SS_DOUBLE','SS_DOUBLE','SS_DOUBLE','SS_DOUBLE','SS_DOUBLE','SS_DOUBLE','SS_DOUBLE','SS_DOUBLE','SS_DOUBLE','SS_DOUBLE','SS_DOUBLE','SS_DOUBLE'}},'OutputPortsLabel',{{'TQI_ACOR','TQ_COR_STAT','SWI_IGK','ACK_TCS','PUC_STAT','F_N_ENG','RLY_AC','F_SUB_TQI','RATIO_TQI_BAS_MAX_STND','VS','TQI','TQFR','N'}},'OutputPortsLabelMode','ON','InputPortsWidth',int32(0),'InputPortsActive',0,'DialogFcn','rtican_message_interface_gui','BlockDisplay',{{'','center'}},'IconTransparency','on','ParameterTunableNames',{{}},'InitLevel',3,'BlockName',struct('Token',{{'L_EMS1'}}),'SampleTime',{{-1}},'TriggerPort',{{'none'}},'EnablePort',{{'none'}})  RTIBlockParameters=struct('BoardTypeNo',{{1,'OFF',[]}},'BoardNo',{{1,'ON',[1 16]}},'ChannelNo',{{1,'ON',[1 2]}},'Parameters',{{struct('DataFileSupport',struct('DataFileSelectedMaster',1,'DataFileSelectedLocal',1,'DataFileName','c:\users\mpc_car\documents\github\mpc-car\controller\dbcfiles\hmc_can_for_ucb_v2.dbc|','DataFileDate',['21-Nov-2014 13:30:51'],'SelectedFile','c:\users\mpc_car\documents\github\mpc-car\dbcfiles\hmc_can_for_ucb_v2.dbc','InterfaceFcn','rtican_dbc_file_parser'),'Options',struct('StatusSelected',0,'TimeSelected',0,'DeltaTimeSelected',0,'BytePortSelected',0,'MessageLengthSelected',0,'TriggerPort',struct('Selected',0,'TriggerType',0),'UserCoding',struct('Selected',0,'InterfaceFile','UserDecodingFile','FcnName','UserDecodeFcn','InportSelected',0,'InportWidth',1,'OutportSelected',0,'OutportWidth',1),'EnablePortSelected',0,'SignalOnPortnameSelected',1,'UseRXService',0),'Message',struct('MsgOnBlocknameSelected',1,'MsgName','L_EMS1','MsgIdFormat',0,'MsgId',514,'MsgLength',8,'NumSignals',13,'SampleTime',-1,'Signal',struct('SgnName',{'TQI_ACOR','TQ_COR_STAT','SWI_IGK','ACK_TCS','PUC_STAT','F_N_ENG','RLY_AC','F_SUB_TQI','RATIO_TQI_BAS_MAX_STND','VS','TQI','TQFR','N'},'SgnStartBit',{0,8,10,11,12,13,14,15,16,24,32,40,48},'SgnLength',{8,2,1,1,1,1,1,1,8,8,8,8,16},'ByteLayout',{0,0,0,0,0,0,0,0,0,0,0,0,0},'Factor',{0.390625,1,1,1,1,1,1,1,0.0078,1,0.390625,0.390625,0.25},'Offset',{0,0,0,0,0,0,0,0,0,0,0,0,0},'SgnComment',{['In case of Delphi ECU, Output period tolerance(+1ms) will be applied to Engine Lamda3.'],['In case of Delphi ECU, Output period tolerance(+1ms) will be applied to Engine Lamda3.'],['In case of Delphi ECU, Output period tolerance(+1ms) will be applied to Engine Lamda3.'],['In case of Delphi ECU, Output period tolerance(+1ms) will be applied to Engine Lamda3.'],['In case of Delphi ECU, Output period tolerance(+1ms) will be applied to Engine Lamda3.'],['In case of Delphi ECU, Output period tolerance(+1ms) will be applied to Engine Lamda3.'],['In case of Delphi ECU, Output period tolerance(+1ms) will be applied to Engine Lamda3.'],['In case of Delphi ECU, Output period tolerance(+1ms) will be applied to Engine Lamda3.'],['In case of Delphi ECU, Output period tolerance(+1ms) will be applied to Engine Lamda3.'],['In case of Delphi ECU, Output period tolerance(+1ms) will be applied to Engine Lamda3.'],['In case of Delphi ECU, Output period tolerance(+1ms) will be applied to Engine Lamda3.'],['In case of Delphi ECU, Output period tolerance(+1ms) will be applied to Engine Lamda3.'],['In case of Delphi ECU, Output period tolerance(+1ms) will be applied to Engine Lamda3.']},'SgnUnit',{'%','','','','','','','','','km/h','%','%','rpm'},'Min',{0,0,0,0,0,0,0,0,0,0,0,0,0},'Max',{99.6094,3,1,1,1,1,1,1,2,255,99.6094,99.6094,16383.75},'SgnType',{0,0,0,0,0,0,0,0,0,0,0,0,0},'SLDataType',{'SS_DOUBLE','SS_DOUBLE','SS_DOUBLE','SS_DOUBLE','SS_DOUBLE','SS_DOUBLE','SS_DOUBLE','SS_DOUBLE','SS_DOUBLE','SS_DOUBLE','SS_DOUBLE','SS_DOUBLE','SS_DOUBLE'},'DataType',{0,0,0,0,0,0,0,0,0,0,0,0,0},'ModeValue',{-1,-1,-1,-1,-1,-1,-1,-1,-1,-1,-1,-1,-1}),'MsgIdNumFormat',0,'MsgComment',{{''}}),'Version',1.2,'general',struct('isFromLib',0)),'OFF',[]}},'GroupId',{{struct('Group',{{'RTICAN'}},'No',1,'Behavior',{{'NAMECHANGE'}},'BlockType',{{'SINK'}},'NameChangeFlag',0),'OFF',[]}},'SFcnRTICANMessage',{{struct('MsgType','RX','SFcnPortType','Scalar','MsgName','L_EMS1','MsgIdFormat','STD','MsgId',514,'MsgLength',8,'NumSignals',13,'SampleTime',-1,'Signal',struct('SgnName',{'TQI_ACOR','TQ_COR_STAT','SWI_IGK','ACK_TCS','PUC_STAT','F_N_ENG','RLY_AC','F_SUB_TQI','RATIO_TQI_BAS_MAX_STND','VS','TQI','TQFR','N'},'SgnStartBit',{0,8,10,11,12,13,14,15,16,24,32,40,48},'SgnLength',{8,2,1,1,1,1,1,1,8,8,8,8,16},'ByteLayout',{['little endian'],['little endian'],['little endian'],['little endian'],['little endian'],['little endian'],['little endian'],['little endian'],['little endian'],['little endian'],['little endian'],['little endian'],['little endian']},'Factor',{0.390625,1,1,1,1,1,1,1,0.0078,1,0.390625,0.390625,0.25},'Offset',{0,0,0,0,0,0,0,0,0,0,0,0,0},'SgnType',{'standard','standard','standard','standard','standard','standard','standard','standard','standard','standard','standard','standard','standard'},'SLDataType',{'SS_DOUBLE','SS_DOUBLE','SS_DOUBLE','SS_DOUBLE','SS_DOUBLE','SS_DOUBLE','SS_DOUBLE','SS_DOUBLE','SS_DOUBLE','SS_DOUBLE','SS_DOUBLE','SS_DOUBLE','SS_DOUBLE'},'DataType',{['unsigned int'],['unsigned int'],['unsigned int'],['unsigned int'],['unsigned int'],['unsigned int'],['unsigned int'],['unsigned int'],['unsigned int'],['unsigned int'],['unsigned int'],['unsigned int'],['unsigned int']},'ModeValue',{-1,-1,-1,-1,-1,-1,-1,-1,-1,-1,-1,-1,-1}),'StatusSelected','no','TimeSelected','no','DeltaTimeSelected','no','BytePortSelected','no','MessageLengthSelected','no','TriggerPort',struct('Selected','no','TriggerType',0),'UserCoding',struct('Selected','no','InterfaceFile','UserDecodingFile','FcnName','UserDecodeFcn','InportSelected','no','InportWidth',1,'OutportSelected','no','OutportWidth',1),'EnablePortSelected','no','UseRXService','no','BoardType','DS1','BoardNo',1,'ControllerNo',1),'OFF',[]}},'TLCFileName',{{'rtican_rx_message','OFF',[]}})  RTISFcnParameters=struct('SFcnRTICANMessage','struct','TLCFileName','char')  RTIBlockParaDefault=struct('BoardTypeNo',4302,'BoardNo',1,'ChannelNo',1,'Parameters',struct('DataFileSupport',struct('DataFileSelectedMaster',0,'DataFileSelectedLocal',0,'DataFileName','','DataFileDate','','SelectedFile',['<no file selected>']),'Options',struct('StatusSelected',1,'TimeSelected',1,'DeltaTimeSelected',1,'BytePortSelected',0,'MessageLengthSelected',0,'TriggerPort',struct('Selected',0,'TriggerType','rising'),'UserCoding',struct('Selected',0,'InterfaceFile','UserDecodingFile','FcnName','UserDecodeFcn','InportSelected',0,'InportWidth',1,'OutportSelected',0,'OutportWidth',1),'EnablePortSelected',0,'SignalOnPortnameSelected',1,'UseRXService',0),'Message',struct('MsgOnBlocknameSelected',0,'MsgName',['RX Message'],'MsgIdFormat',0,'MsgId',100,'MsgLength',8,'NumSignals',1,'SampleTime',-1,'Signal',struct('SgnName',['RX signal'],'SgnStartBit',0,'SgnLength',8,'SgnType',0,'ModeValue',-1,'DataType',0,'SLDataType','SS_DOUBLE','ByteLayout',0,'Factor',1,'Offset',0,'Min',0,'Max',255,'SgnComment',{{}},'SgnUnit',''),'MsgIdNumFormat',0,'MsgComment',{{''}}),'Version',1.2,'general',struct('isFromLib',1)),'GroupId',struct('Group',{{'RTICAN'}},'No',1,'Behavior',{{'NAMECHANGE'}},'BlockType',{{'SINK'}},'NameChangeFlag',0),'SFcnRTICANMessage',struct('MsgType','RX','MsgName',['RX Message'],'MsgIdFormat','STD','MsgId',100,'MsgLength',8,'NumSignals',1,'SampleTime',-1,'Signal',struct('SgnName',['RX signal'],'SgnStartBit',0,'SgnLength',8,'SgnType','standard','ModeValue',-1,'DataType',['unsigned int'],'ByteLayout',['little endian'],'SLDataType','SS_DOUBLE','Factor',1,'Offset',0),'StatusSelected','yes','TimeSelected','yes','DeltaTimeSelected','yes','BytePortSelected','no','MessageLengthSelected','no','EnablePortSelected','no','UserCoding',struct('Selected','no','InterfaceFile','UserDecodingFile','FcnName','UserDecodeFcn','InportSelected','no','InportWidth',1,'OutportSelected','no','OutportWidth',1),'TriggerPort',struct('Selected','no','TriggerType','rising'),'UseRXService','no','BoardType','DS4302','BoardNo',1,'ControllerNo',1,'SFcnPortType','Scalar'),'TLCFileName','rtican_rx_message')
      settings: AttributesFormatString=Group Id: RTICAN1\n
  EMS1_CAN : Outport
  wires:
  Bus Creator/1 -> EMS1_CAN/1  "EMS1_CAN"
  L_EMS1/1 -> Bus Creator/1  "TQI_ACOR"
  L_EMS1/2 -> Bus Creator/2  "TQ_COR_STAT"
  L_EMS1/3 -> Bus Creator/3  "SWI_IGK"
  L_EMS1/4 -> Bus Creator/4  "ACK_TCS"
  L_EMS1/5 -> Bus Creator/5  "PUC_STAT"
  L_EMS1/6 -> Bus Creator/6  "F_N_ENG"
  L_EMS1/7 -> Bus Creator/7  "RLY_AC"
  L_EMS1/8 -> Bus Creator/8  "F_SUB_TQI"
  L_EMS1/9 -> Bus Creator/9  "RATIO_TQI_BAS_MAX_STND"
  L_EMS1/10 -> Bus Creator/10  "VS"
  L_EMS1/11 -> Bus Creator/11  "TQI"
  L_EMS1/12 -> Bus Creator/12  "TQFR"
  L_EMS1/13 -> Bus Creator/13  "N"

== system Control_test/InputProcessing/VehicleCanProcessing/EMS1Processing ==
  In1 : Inport
  In2 : Inport  Port=2
  Bus Creator : BusCreator  Inputs=5
  Bus Selector1 : BusSelector  OutputSignals=TQ_STND,BRAKE_ACT
  Bus Selector3 : BusSelector  OutputSignals=VS,TQFR,TQI
  EMS1 Processing : Subsystem
  Gain : Gain  Gain=1/100
  Product : Product  RndMeth=Zero
  Terminator : Terminator
  out1 : Outport
  wires:
  EMS1 Processing/2(ipEmsVehSpdFail) -> Terminator/1
  In1/1 -> Bus Selector3/1
  Bus Selector3/1 -> EMS1 Processing/1(VS_CAN)  "<VS>"
  In2/1 -> Bus Selector1/1
  Bus Selector3/3 -> Product/1  "<TQI>"
  Bus Selector1/1 -> Product/2, Bus Creator/4  "<TQ_STND>"
  Bus Creator/1 -> out1/1  "EMS1"
  EMS1 Processing/1(ipEmsVehSpd [kph]) -> Bus Creator/1
  Bus Selector3/2 -> Bus Creator/2  "<TQFR>"
  Product/1 -> Gain/1  "Engine_Torque"
  Bus Selector1/2 -> Bus Creator/5  "<BRAKE_ACT>"
  Gain/1 -> Bus Creator/3  "Engine_Torque"
